simulink model "FuzzyControl"  (Simulink 8.5)
settings: Solver=ode45  StartTime=0.0  StopTime=2500  RelTol=1e-3
libraries: fuzblock x1
settings Model: Creator=YH  LastModifiedBy=YH
settings DataIOCC: SignalLoggingSaveFormat=Dataset
settings OptimizationCC: ExpressionDepthLimit=128
settings DebuggingCC: UnderspecifiedInitializationDetection=Simplified  MergeDetectMultiDrivingBlocksExec=error  FcnCallInpInsideContextMsg=EnableAllAsError  StateNameClashWarn=none
settings GRTTargetCC: CombineOutputUpdateFcns=on  GRTInterface=off

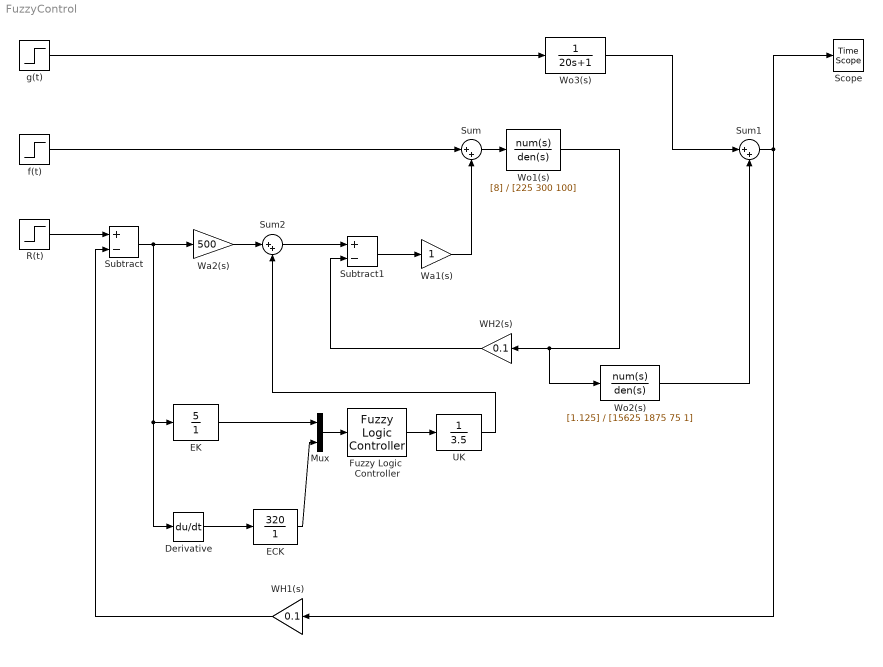
== system FuzzyControl ==
  Derivative : Derivative
  "ECK " : TransferFcn  Numerator=[320]  Denominator=[1]
  EK : TransferFcn  Numerator=[5]  Denominator=[1]
  Fuzzy Logic  Controller : fuzblock/Fuzzy Logic  Controller  RequirementInfo={} %GIDa_a8036bfa_e616_4cd4_b504_79abde121963  fis=fuzzyController
  Mux : Mux  Inputs=2
  R(t) : Step  SampleTime=0
  Scope : TimeScope
  Subtract : Sum  Inputs=+-
  Subtract1 : Sum  Inputs=+-
  Sum : Sum  Inputs=|++
  Sum1 : Sum  Inputs=|++
  Sum2 : Sum  Inputs=|++
  UK : TransferFcn  Denominator=[3.5]
  WH1(s) : Gain  Gain=0.1
  WH2(s) : Gain  Gain=0.1
  Wa1(s) : Gain
  Wa2(s) : Gain  Gain=500
  Wo1(s) : TransferFcn  Numerator=[8]  Denominator=[225 300 100]
  Wo2(s) : TransferFcn  Numerator=[1.125]  Denominator=[15625 1875 75 1]
  Wo3(s) : TransferFcn  Denominator=[20 1]
  f(t) : Step  Time=500  After=10  SampleTime=0
  g(t) : Step  Time=300  After=10  SampleTime=0
  wires:
  R(t)/1 -> Subtract/1
  WH1(s)/1 -> Subtract/2
  Sum1/1 -> Scope/1, WH1(s)/1
  g(t)/1 -> Wo3(s)/1
  Wo3(s)/1 -> Sum1/1
  Wo1(s)/1 -> Wo2(s)/1, WH2(s)/1
  Wo2(s)/1 -> Sum1/2
  Sum/1 -> Wo1(s)/1
  f(t)/1 -> Sum/1
  Wa1(s)/1 -> Sum/2
  Subtract1/1 -> Wa1(s)/1
  WH2(s)/1 -> Subtract1/2
  Derivative/1 -> "ECK "/1
  Mux/1 -> Fuzzy Logic  Controller/1
  Fuzzy Logic  Controller/1 -> UK/1
  EK/1 -> Mux/1
  "ECK "/1 -> Mux/2
  Subtract/1 -> Wa2(s)/1, Derivative/1, EK/1
  UK/1 -> Sum2/2
  Sum2/1 -> Subtract1/1
  Wa2(s)/1 -> Sum2/1
